simulink model "tutorial_simulink_2"  (R2024b)
settings: Solver=VariableStepAuto  StartTime=0.0  StopTime=10.0  RelTol=1e-3
settings Model: Creator=user  LastModifiedBy=user

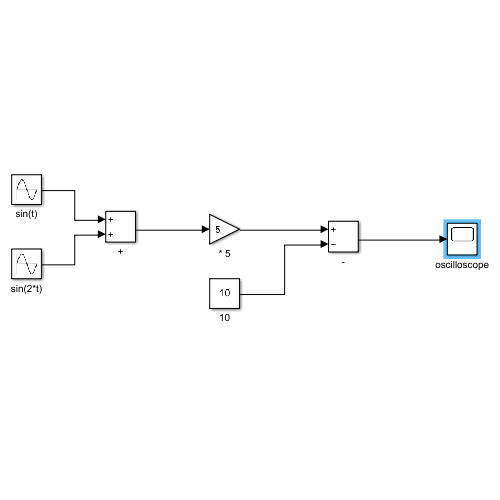
[thumbnail: Simulink's stored preview of the top-level diagram]
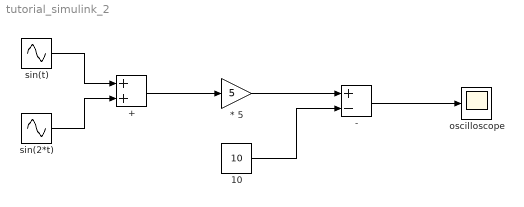
== system tutorial_simulink_2 ==
  * 5 : Gain  Gain=5
  + : Sum
  - : Sum  Inputs=+-
  10 : Constant  Value=10
  oscilloscope : Scope
  sin(2*t) : Sin  Frequency=2  SampleTime=0
  sin(t) : Sin  SampleTime=0
  wires:
  sin(t)/1 -> +/1
  sin(2*t)/1 -> +/2
  +/1 -> * 5/1
  * 5/1 -> -/1
  -/1 -> oscilloscope/1
  10/1 -> -/2
